simulink model "Problem3"  (R2020b)
settings: Solver=VariableStepAuto  StartTime=0.0  StopTime=10.0  RelTol=1e-3
undefined symbols (not defined in the file or in its folder): b, m
settings Model: DataDictionary=NewData.sldd  Creator=Dell  LastModifiedBy=Dell

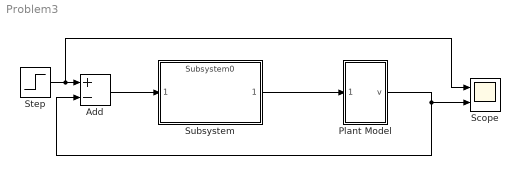
== system Problem3 ==
  Add : Sum  Inputs=+-
  Plant Model : Subsystem
  Scope : Scope  NumInputPorts=2
  Step : Step  SampleTime=0
  Subsystem : ModelReference  ModelNameDialog=Subsystem0  SimulationMode=Normal  ModelReferenceVersion=1.2
  wires:
  Subsystem/1 -> Plant Model/1(Outport)
  Plant Model/1(v) -> Add/2, Scope/2
  Add/1 -> Subsystem/1
  Step/1 -> Scope/1, Add/1

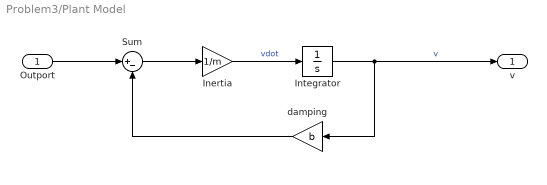
== system Problem3/Plant Model ==
  Outport : Inport
  Inertia : Gain  Gain=1/m
  Integrator : Integrator
  Sum : Sum  Inputs=|+-
  damping : Gain  Gain=b
  v : Outport
  wires:
  Inertia/1 -> Integrator/1  "vdot"
  Integrator/1 -> v/1, damping/1  "v"
  damping/1 -> Sum/2
  Sum/1 -> Inertia/1
  Outport/1 -> Sum/1
